simulink model "ar_lht_hw"  (R2018a)
settings: Solver=VariableStepAuto  StartTime=0.0  StopTime=ts*2+2*maxRho*T*2  RelTol=1e-3  EnableMultiTasking=on
PreLoadFcn:
  | currentDir  = pwd;
  | filesepIdx   = strfind(currentDir, filesep);
  | newDir = currentDir(1:filesepIdx(end)-7);
  | 
  | addpath([newDir, '\scripts']);
InitFcn:
  | setup;
  | pre_processing;
StopFcn:
  | post_processing;
  | imtool(O);
values from neighbouring files (symbols this model uses):
  deltaTheta = 1    [setup.m]
  fps = f/((height)*(width))    (= 184.377034505)    [setup.m]
  height = 768    [setup.m]
  K = (maxTheta + deltaTheta)/R    (= 45)    [setup.m]
  maxRho = ceil(sqrt((height/2)^2+(width/2)^2))    [setup.m]
  maxTheta = 179    [setup.m]
  R = 4    [setup.m]
  T = 1/f    (= 6.89655172414e-09)    [setup.m]
  width = 1024    [setup.m]
libraries: xbsIndex_r4 x336, hdlsllib x6, visionhdlutilities x2, visionhdlio x2, simulink x1, dspswit3 x1, visionsources x1
(part 1 of 2)
settings Model: Creator=David Northcote  LastModifiedBy=rgb11127
settings OptimizationCC: LifeSpan=inf
settings DebuggingCC: SFUnexpectedBacktrackingDiag=warning  SFNoUnconditionalDefaultTransitionDiag=warning  SFExecutionAtInitializationDiag=none
settings CodeAppCC: StateflowObjectComments=on
settings GRTTargetCC: TargetLangStandard=C89/C90 (ANSI)  GeneratePreprocessorConditionals=Disable all
settings ConfigComp: CovMetricSettings=dw  CovHtmlReporting=on  CovSaveCumulativeToWorkspaceVar=on  CovSaveSingleToWorkspaceVar=on  CovExternalEMLEnable=off

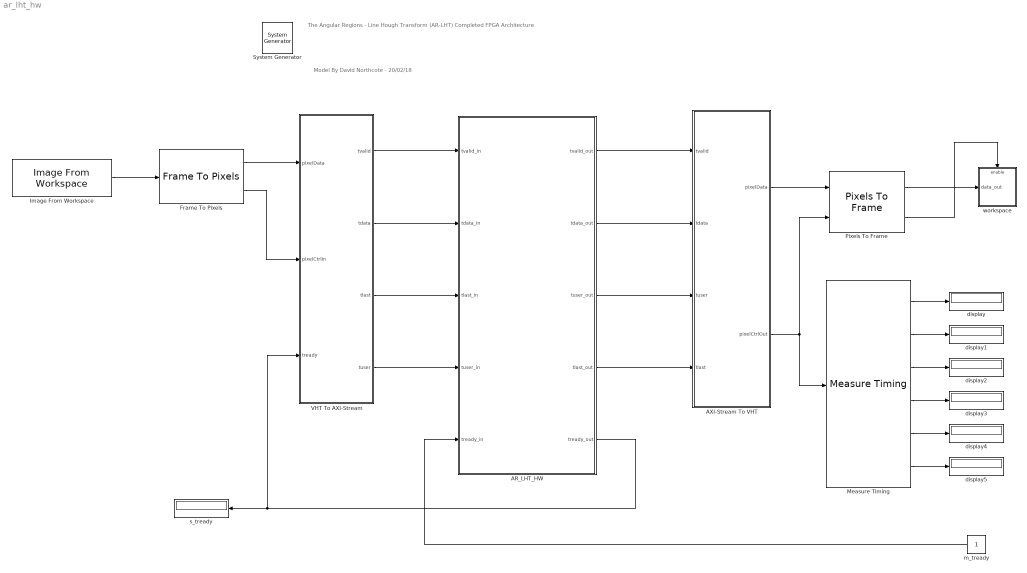
== system ar_lht_hw ==
  note: Model By David Northcote - 20/02/18
  note: The Angular Regions - Line Hough Transform (AR-LHT)
      | Completed FPGA Architecture
  " System Generator" : xbsIndex_r4/ System Generator  Tag=genX  xilinxfamily=zynq  part=xc7z010  speed=-1  package=clg400  synthesis_tool=Vivado  clock_wrapper=Clock Enables  directory=./netlist  proj_type=Vivado  Synth_file=Vivado Synthesis Defaults  Impl_file=Vivado Implementation Defaults  testbench=off  simulink_period=T  sysclk_period=T*1e9  dcm_input_clock_period=10  incr_netlist=off  trim_vbits=Everywhere in SubSystem  dbl_ovrd=According to Block Masks  core_generation=According to Block Masks  run_coregen=off  deprecated_control=off  eval_field=0  block_type=sysgen
  AR_LHT_HW : Subsystem
  AXI-Stream To VHT : Subsystem
  Frame To Pixels : visionhdlio/Frame To Pixels  NumComponents=1  VideoFormat=Custom  ActivePixelsPerLine=width  ActiveVideoLines=height  TotalPixelsPerLine=width  TotalVideoLines=height  StartingActiveLine=1  FrontPorch=0  SampleTime=0
      settings: SourceProductName=Vision HDL Toolbox  SourceProductBaseCode=VT
  Image From Workspace : visionsources/Image From Workspace  Tag=vipblks_nd  ImageValue=InputImage  Ts=1/fps  imagePorts=One multidimensional signal  OutPortLabels=R|G|B  ImageDataType=Inherit from 'Value'  Signed=on  WordLength=16  sdImageDataType=sfix(16)  FractionLengthMode=User-defined  FractionLength=15
      settings: SourceProductName=Computer Vision System Toolbox  SourceProductBaseCode=VP
  Measure Timing : visionhdlutilities/Measure Timing  SimulateUsing=Code generation
      settings: SourceProductName=Vision HDL Toolbox  SourceProductBaseCode=VT
  Pixels To Frame : visionhdlio/Pixels To Frame  NumComponents=1  VideoFormat=Custom  ActivePixelsPerLine=maxRho*2  ActiveVideoLines=maxTheta+deltaTheta  TotalPixelsPerLine=maxRho*2  TotalVideoLines=maxTheta+deltaTheta
      settings: SourceProductName=Vision HDL Toolbox  SourceProductBaseCode=VT
  VHT To AXI-Stream : Subsystem
  display{,1..5} (6 alike) : Display
  m_tready : Constant  OutDataTypeStr=boolean  SampleTime=T
  s_tready : Display
  workspace : Subsystem
  wires:
  Measure Timing/6 -> display5/1
  Measure Timing/5 -> display4/1
  Measure Timing/4 -> display3/1
  Measure Timing/3 -> display2/1
  Measure Timing/2 -> display1/1
  Measure Timing/1 -> display/1
  Pixels To Frame/2 -> workspace/Enable
  Pixels To Frame/1 -> workspace/1(data_out)
  AXI-Stream To VHT/2(pixelCtrlOut) -> Measure Timing/1, Pixels To Frame/2
  AXI-Stream To VHT/1(pixelData) -> Pixels To Frame/1
  Image From Workspace/1 -> Frame To Pixels/1
  Frame To Pixels/2 -> VHT To AXI-Stream/2(pixelCtrlIn)
  Frame To Pixels/1 -> VHT To AXI-Stream/1(pixelData)
  VHT To AXI-Stream/4(tuser) -> AR_LHT_HW/4(tuser_in)
  VHT To AXI-Stream/2(tdata) -> AR_LHT_HW/2(tdata_in)
  VHT To AXI-Stream/3(tlast) -> AR_LHT_HW/3(tlast_in)
  VHT To AXI-Stream/1(tvalid) -> AR_LHT_HW/1(tvalid_in)
  AR_LHT_HW/5(tready_out) -> VHT To AXI-Stream/3(tready), s_tready/1
  AR_LHT_HW/1(tvalid_out) -> AXI-Stream To VHT/1(tvalid)
  AR_LHT_HW/2(tdata_out) -> AXI-Stream To VHT/2(tdata)
  AR_LHT_HW/3(tuser_out) -> AXI-Stream To VHT/3(tuser)
  AR_LHT_HW/4(tlast_out) -> AXI-Stream To VHT/4(tlast)
  m_tready/1 -> AR_LHT_HW/5(tready_in)

== system ar_lht_hw/AR_LHT_HW ==
  tvalid_in : Inport
  tdata_in : Inport  Port=2
  tlast_in : Inport  Port=3
  tuser_in : Inport  Port=4
  tready_in : Inport  Port=5
  DUT : Subsystem
  M_AXIS : Subsystem
  S_AXIS : Subsystem
  tvalid_out : Outport
  tdata_out : Outport  Port=2
  tuser_out : Outport  Port=3
  tlast_out : Outport  Port=4
  tready_out : Outport  Port=5
  wires:
  tdata_in/1 -> S_AXIS/2(tdata_in)
  tuser_in/1 -> S_AXIS/4(tuser_in)
  tvalid_in/1 -> S_AXIS/1(tvalid_in)
  tlast_in/1 -> S_AXIS/3(tlast_in)
  M_AXIS/2(tvalid_out) -> tvalid_out/1
  tready_in/1 -> M_AXIS/5(tready_in)
  M_AXIS/3(tdata_out) -> tdata_out/1
  M_AXIS/5(tlast_out) -> tlast_out/1
  S_AXIS/5(tready_out) -> tready_out/1
  M_AXIS/4(tuser_out) -> tuser_out/1
  S_AXIS/4(tuser_out) -> DUT/4(tuser_in)
  S_AXIS/3(tlast_out) -> DUT/3(tlast_in)
  S_AXIS/1(tvalid_out) -> DUT/1(tvalid_in)
  S_AXIS/2(tdata_out) -> DUT/2(tdata_in)
  DUT/4(tuser_out) -> M_AXIS/4(tuser_in)
  DUT/3(tlast_out) -> M_AXIS/3(tlast_in)
  DUT/2(tdata_out) -> M_AXIS/2(tdata_in)
  DUT/1(tvalid_out) -> M_AXIS/1(tvalid_in)
  M_AXIS/1(tready_out) -> DUT/5(tready_in)
  DUT/5(tready_out) -> S_AXIS/5(tready_in)

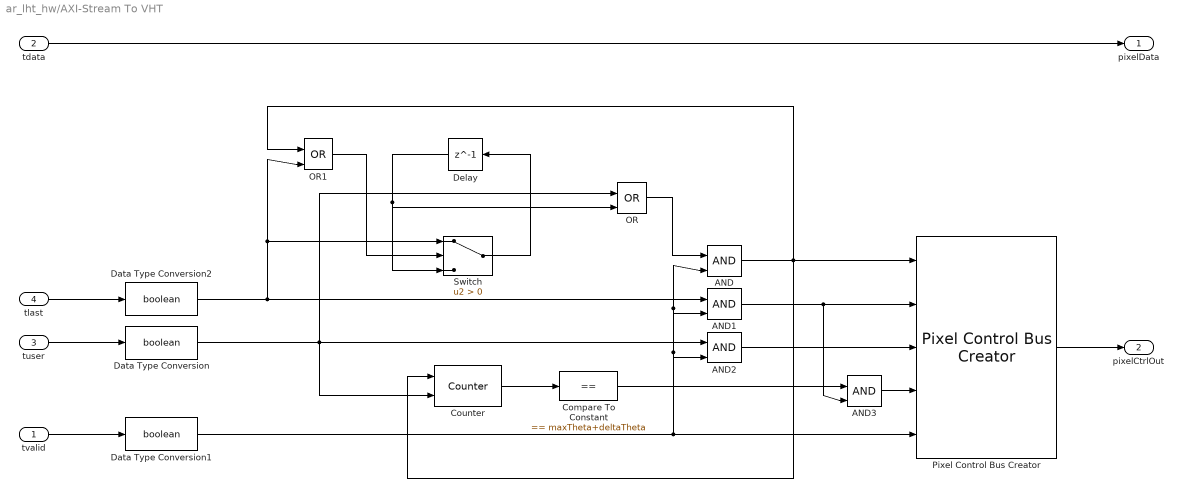
== system ar_lht_hw/AXI-Stream To VHT ==
  tvalid : Inport
  tdata : Inport  Port=2
  tuser : Inport  Port=3
  tlast : Inport  Port=4
  AND{,1..3} (4 alike) : Logic  IconShape=distinctive  AllPortsSameDT=off  OutDataTypeStr=boolean
  Compare To Constant : simulink/Logic and Bit Operations/Compare To Constant  relop===  const=maxTheta+deltaTheta  OutDataTypeStr=boolean
  Counter : dspswit3/Counter  Direction=Up  CountEvent=Non-zero sample  CounterSize=32 bits  MaxCount=255  InitialCount=0  Output=Count  HitValue=32  ResetInput=on  SamplesPerFrame=1  Ts=1  CntDtype=uint32  HitDtype=Logical
  Data Type Conversion : DataTypeConversion  OutDataTypeStr=boolean
  Data Type Conversion1 : DataTypeConversion  OutDataTypeStr=boolean
  Data Type Conversion2 : DataTypeConversion  OutDataTypeStr=boolean
  Delay : Delay  DelayLength=1
  OR : Logic  Operator=OR  IconShape=distinctive  AllPortsSameDT=off  OutDataTypeStr=boolean
  OR1 : Logic  Operator=OR  IconShape=distinctive  AllPortsSameDT=off  OutDataTypeStr=boolean
  Pixel Control Bus Creator : visionhdlutilities/Pixel Control Bus Creator
      settings: SourceProductName=Vision HDL Toolbox  SourceProductBaseCode=VT
  Switch : Switch  Criteria=u2 > Threshold
  pixelData : Outport
  pixelCtrlOut : Outport  Port=2
  wires:
  AND3/1 -> Pixel Control Bus Creator/4
  AND1/1 -> Pixel Control Bus Creator/2, AND3/2
  Compare To Constant/1 -> AND3/1
  AND2/1 -> Pixel Control Bus Creator/3
  AND/1 -> Pixel Control Bus Creator/1, OR1/1, Counter/1
  OR1/1 -> Switch/2
  Delay/1 -> Switch/3, OR/2
  Switch/1 -> Delay/1
  OR/1 -> AND/1
  Data Type Conversion/1 -> OR/1, AND2/1, Counter/2
  Data Type Conversion1/1 -> Pixel Control Bus Creator/5, AND/2, AND1/2, AND2/2
  Data Type Conversion2/1 -> Switch/1, OR1/2, AND1/1
  Counter/1 -> Compare To Constant/1
  tvalid/1 -> Data Type Conversion1/1
  tlast/1 -> Data Type Conversion2/1
  tuser/1 -> Data Type Conversion/1
  Pixel Control Bus Creator/1 -> pixelCtrlOut/1
  tdata/1 -> pixelData/1

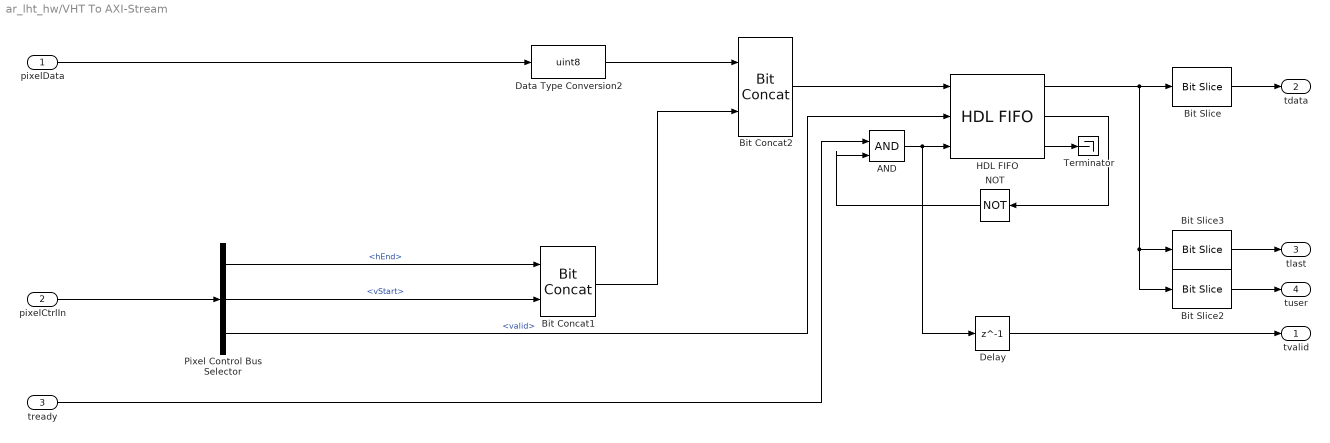
== system ar_lht_hw/VHT To AXI-Stream ==
  pixelData : Inport
  pixelCtrlIn : Inport  Port=2
  tready : Inport  Port=3
  AND : Logic  IconShape=distinctive  AllPortsSameDT=off  OutDataTypeStr=boolean
  Bit Concat1 : hdlsllib/Logic and Bit Operations/Bit Concat  numInputs=2
      settings: SourceProductName=HDL Coder  SourceProductBaseCode=HD
  Bit Concat2 : hdlsllib/Logic and Bit Operations/Bit Concat  numInputs=2
      settings: SourceProductName=HDL Coder  SourceProductBaseCode=HD
  Bit Slice : hdlsllib/Logic and Bit Operations/Bit Slice  lidx=9  ridx=2
  Bit Slice2 : hdlsllib/Logic and Bit Operations/Bit Slice  lidx=0  ridx=0
  Bit Slice3 : hdlsllib/Logic and Bit Operations/Bit Slice  lidx=1  ridx=1
  Data Type Conversion2 : DataTypeConversion  OutDataTypeStr=uint8
  Delay : Delay  DelayLength=1
  HDL FIFO : hdlsllib/HDL RAMs/HDL FIFO  fifo_size=1024  ratio=1  push_msg=Error  pop_msg=Error  show_empty=on  show_full=on  show_num=off
      settings: SourceProductName=HDL Coder  SourceProductBaseCode=HD
  NOT : Logic  Operator=NOT  IconShape=distinctive  AllPortsSameDT=off  OutDataTypeStr=boolean
  Pixel Control Bus Selector : BusSelector  OutputSignals=hEnd,vStart,valid
  Terminator : Terminator
  tvalid : Outport
  tdata : Outport  Port=2
  tlast : Outport  Port=3
  tuser : Outport  Port=4
  wires:
  HDL FIFO/3 -> Terminator/1
  Delay/1 -> tvalid/1
  Pixel Control Bus Selector/3 -> HDL FIFO/2  "<valid>"
  Pixel Control Bus Selector/2 -> Bit Concat1/2  "<vStart>"
  Pixel Control Bus Selector/1 -> Bit Concat1/1  "<hEnd>"
  AND/1 -> HDL FIFO/3, Delay/1
  Bit Slice2/1 -> tuser/1
  Bit Slice3/1 -> tlast/1
  Bit Slice/1 -> tdata/1
  NOT/1 -> AND/2
  HDL FIFO/2 -> NOT/1
  tready/1 -> AND/1
  HDL FIFO/1 -> Bit Slice/1, Bit Slice2/1, Bit Slice3/1
  Bit Concat1/1 -> Bit Concat2/2
  Data Type Conversion2/1 -> Bit Concat2/1
  Bit Concat2/1 -> HDL FIFO/1
  pixelCtrlIn/1 -> Pixel Control Bus Selector/1
  pixelData/1 -> Data Type Conversion2/1

== system ar_lht_hw/workspace ==
  data_out : Inport
  Enable : EnablePort
  To Workspace : ToWorkspace  VariableName=data_out  SampleTime=-1
      settings: MaxDataPoints=1
  wires:
  data_out/1 -> To Workspace/1

== system ar_lht_hw/AR_LHT_HW/DUT ==
  tvalid_in : Inport
  tdata_in : Inport  Port=2
  tlast_in : Inport  Port=3
  tuser_in : Inport  Port=4
  tready_in : Inport  Port=5
  AXI FIFO : xbsIndex_r4/AXI FIFO  input_depth_axis=16  actual_fifo_depth_label=18  enable_tdata=on  enable_tdest=off  enable_tstrb=off  enable_tready=on  enable_tid=off  enable_tuser=on  enable_tkeep=off  enable_tlast=on  has_aresetn=off  enable_data_counts_axis=off  fifo_implementation_type_axis=Common Clock Distributed RAM  trim_axipin_name=on  programmable_full_type_axis=Full  full_threshold_assert_value_axis=0  programmable_empty_type_axis=Empty  empty_threshold_assert_value_axis=1022  underflow_flag_axi=0  underflow_sense_axi=Active High  overflow_flag_axi=0  overflow_sense_axi=Active High  block_type=axi_fifo
  Algorithm : Subsystem
  tvalid_out : Outport
  tdata_out : Outport  Port=2
  tlast_out : Outport  Port=3
  tuser_out : Outport  Port=4
  tready_out : Outport  Port=5
  wires:
  Algorithm/1(tready_out) -> AXI FIFO/1
  Algorithm/2(tvalid_out) -> AXI FIFO/2
  Algorithm/3(tdata_out) -> AXI FIFO/3
  Algorithm/4(tlast_out) -> AXI FIFO/4
  Algorithm/5(tuser_out) -> AXI FIFO/5
  AXI FIFO/5 -> tready_out/1
  AXI FIFO/2 -> tdata_out/1
  AXI FIFO/1 -> tvalid_out/1
  AXI FIFO/3 -> tlast_out/1
  AXI FIFO/4 -> tuser_out/1
  tdata_in/1 -> Algorithm/3(tdata_in)
  tuser_in/1 -> Algorithm/5(tuser_in)
  tlast_in/1 -> Algorithm/4(tlast_in)
  tready_in/1 -> Algorithm/1(tready_in)
  tvalid_in/1 -> Algorithm/2(tvalid_in)

== system ar_lht_hw/AR_LHT_HW/M_AXIS ==
  tvalid_in : Inport
  tdata_in : Inport  Port=2
  tlast_in : Inport  Port=3
  tuser_in : Inport  Port=4
  tready_in : Inport  Port=5
  m_axis_tdata : xbsIndex_r4/Gateway Out  inherit_from_input=on  hdl_port=on  rows=1  columns=1  UseAsDAC=off  DACChannel='1'  interface=None  automatic_assignment=on  address_offset=hex2dec('00')  intf_name=''  intf_description=''  timing_constraint=None  locs_specified=off  LOCs={}  io_standard={}  block_type=gatewayout
  m_axis_tlast : xbsIndex_r4/Gateway Out  inherit_from_input=off  hdl_port=on  rows=1  columns=1  UseAsDAC=off  DACChannel='1'  interface=None  automatic_assignment=on  address_offset=hex2dec('00')  intf_name=''  intf_description=''  timing_constraint=None  locs_specified=off  LOCs={}  io_standard={}  block_type=gatewayout
  m_axis_tready : xbsIndex_r4/Gateway In  gui_display_data_type=Boolean  arith_type=Boolean  n_bits=16  bin_pt=14  preci_type=Single  exp_width=8  frac_width=24  rows=1  columns=1  quantization="Round  (unbiased: +/- Inf)"  overflow=Saturate  period=T  UseAsADC=off  ADCChannel='1'  interface=None  automatic_assignment=on  address_offset=hex2dec('00')  intf_name=''  intf_description=''  default_value=0  timing_constraint=None  locs_specified=off  LOCs={}  io_standard={}  inherit_from_input=off  hdl_port=on  dbl_ovrd=off  block_type=gatewayin
  m_axis_tuser : xbsIndex_r4/Gateway Out  inherit_from_input=off  hdl_port=on  rows=1  columns=1  UseAsDAC=off  DACChannel='1'  interface=None  automatic_assignment=on  address_offset=hex2dec('00')  intf_name=''  intf_description=''  timing_constraint=None  locs_specified=off  LOCs={}  io_standard={}  block_type=gatewayout
  m_axis_tvalid : xbsIndex_r4/Gateway Out  inherit_from_input=off  hdl_port=on  rows=1  columns=1  UseAsDAC=off  DACChannel='1'  interface=None  automatic_assignment=on  address_offset=hex2dec('00')  intf_name=''  intf_description=''  timing_constraint=None  locs_specified=off  LOCs={}  io_standard={}  block_type=gatewayout
  tready_out : Outport
  tvalid_out : Outport  Port=2
  tdata_out : Outport  Port=3
  tuser_out : Outport  Port=4
  tlast_out : Outport  Port=5
  wires:
  m_axis_tuser/1 -> tuser_out/1
  m_axis_tvalid/1 -> tvalid_out/1
  m_axis_tdata/1 -> tdata_out/1
  tready_in/1 -> m_axis_tready/1
  tvalid_in/1 -> m_axis_tvalid/1
  m_axis_tlast/1 -> tlast_out/1
  tdata_in/1 -> m_axis_tdata/1
  tlast_in/1 -> m_axis_tlast/1
  m_axis_tready/1 -> tready_out/1
  tuser_in/1 -> m_axis_tuser/1

== system ar_lht_hw/AR_LHT_HW/S_AXIS ==
  tvalid_in : Inport
  tdata_in : Inport  Port=2
  tlast_in : Inport  Port=3
  tuser_in : Inport  Port=4
  tready_in : Inport  Port=5
  s_axis_tdata : xbsIndex_r4/Gateway In  gui_display_data_type=Fixed-point  arith_type=Unsigned  n_bits=8  bin_pt=0  preci_type=Single  exp_width=8  frac_width=24  rows=1  columns=1  quantization=Truncate  overflow=Flag as error  period=T  UseAsADC=off  ADCChannel='1'  interface=None  automatic_assignment=on  address_offset=hex2dec('00')  intf_name=''  intf_description=''  default_value=0  timing_constraint=None  locs_specified=off  LOCs={}  io_standard={}  inherit_from_input=off  hdl_port=on  dbl_ovrd=off  block_type=gatewayin
  s_axis_tlast : xbsIndex_r4/Gateway In  gui_display_data_type=Boolean  arith_type=Boolean  n_bits=32  bin_pt=0  preci_type=Single  exp_width=8  frac_width=24  rows=1  columns=1  quantization=Truncate  overflow=Flag as error  period=T  UseAsADC=off  ADCChannel='1'  interface=None  automatic_assignment=on  address_offset=hex2dec('00')  intf_name=''  intf_description=''  default_value=0  timing_constraint=None  locs_specified=off  LOCs={}  io_standard={}  inherit_from_input=off  hdl_port=on  dbl_ovrd=off  block_type=gatewayin
  s_axis_tready : xbsIndex_r4/Gateway Out  inherit_from_input=on  hdl_port=on  rows=1  columns=1  UseAsDAC=off  DACChannel='1'  interface=None  automatic_assignment=on  address_offset=hex2dec('00')  intf_name=''  intf_description=''  timing_constraint=None  locs_specified=off  LOCs={}  io_standard={}  block_type=gatewayout
  s_axis_tuser : xbsIndex_r4/Gateway In  gui_display_data_type=Boolean  arith_type=Boolean  n_bits=1  bin_pt=0  preci_type=Single  exp_width=8  frac_width=24  rows=1  columns=1  quantization=Truncate  overflow=Flag as error  period=T  UseAsADC=off  ADCChannel='1'  interface=None  automatic_assignment=on  address_offset=hex2dec('00')  intf_name=''  intf_description=''  default_value=0  timing_constraint=None  locs_specified=off  LOCs={}  io_standard={}  inherit_from_input=off  hdl_port=on  dbl_ovrd=off  block_type=gatewayin
  s_axis_tvalid : xbsIndex_r4/Gateway In  gui_display_data_type=Boolean  arith_type=Boolean  n_bits=32  bin_pt=0  preci_type=Single  exp_width=8  frac_width=24  rows=1  columns=1  quantization=Truncate  overflow=Flag as error  period=T  UseAsADC=off  ADCChannel='1'  interface=None  automatic_assignment=on  address_offset=hex2dec('00')  intf_name=''  intf_description=''  default_value=0  timing_constraint=None  locs_specified=off  LOCs={}  io_standard={}  inherit_from_input=off  hdl_port=on  dbl_ovrd=off  block_type=gatewayin
  tvalid_out : Outport
  tdata_out : Outport  Port=2
  tlast_out : Outport  Port=3
  tuser_out : Outport  Port=4
  tready_out : Outport  Port=5
  wires:
  s_axis_tready/1 -> tready_out/1
  tready_in/1 -> s_axis_tready/1
  tuser_in/1 -> s_axis_tuser/1
  tlast_in/1 -> s_axis_tlast/1
  tvalid_in/1 -> s_axis_tvalid/1
  tdata_in/1 -> s_axis_tdata/1
  s_axis_tvalid/1 -> tvalid_out/1
  s_axis_tdata/1 -> tdata_out/1
  s_axis_tlast/1 -> tlast_out/1
  s_axis_tuser/1 -> tuser_out/1

== system ar_lht_hw/AR_LHT_HW/DUT/Algorithm ==
  note: tready should never have any latency. It will only be used to pop the IP core's front-end FIFO.
  tready_in : Inport
  tvalid_in : Inport  Port=2
  tdata_in : Inport  Port=3
  tlast_in : Inport  Port=4
  tuser_in : Inport  Port=5
  AlgorithmDUT_ARHough : Subsystem
  AlgorithmDUT_Open : Subsystem
  tready_out : Outport
  tvalid_out : Outport  Port=2
  tdata_out : Outport  Port=3
  tlast_out : Outport  Port=4
  tuser_out : Outport  Port=5
  wires:
  tready_in/1 -> tready_out/1
  tvalid_in/1 -> AlgorithmDUT_ARHough/4(tvalid_in)
  tuser_in/1 -> AlgorithmDUT_ARHough/1(tuser_in)
  tlast_in/1 -> AlgorithmDUT_ARHough/2(tlast_in)
  tdata_in/1 -> AlgorithmDUT_ARHough/3(tdata_in)
  AlgorithmDUT_ARHough/1(tuser_out) -> AlgorithmDUT_Open/1(tuser_in)
  AlgorithmDUT_ARHough/2(tlast_out) -> AlgorithmDUT_Open/2(tlast_in)
  AlgorithmDUT_ARHough/3(tdata_out) -> AlgorithmDUT_Open/3(tdata_in)
  AlgorithmDUT_ARHough/4(tvalid_out) -> AlgorithmDUT_Open/4(tvalid_in)
  AlgorithmDUT_Open/1(tuser_out) -> tuser_out/1
  AlgorithmDUT_Open/2(tlast_out) -> tlast_out/1
  AlgorithmDUT_Open/3(tdata_out) -> tdata_out/1
  AlgorithmDUT_Open/4(tvalid_out) -> tvalid_out/1

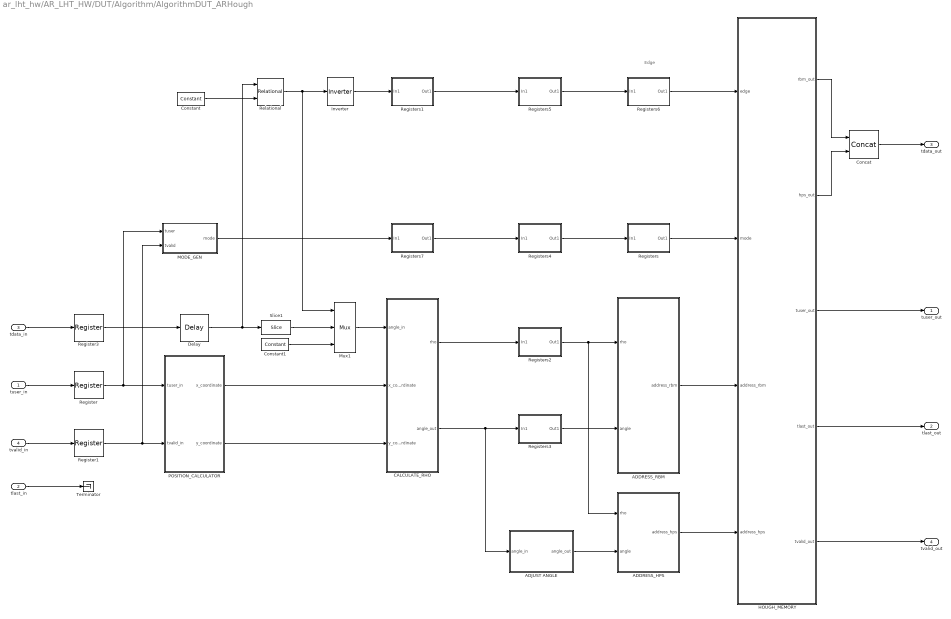
== system ar_lht_hw/AR_LHT_HW/DUT/Algorithm/AlgorithmDUT_ARHough ==
  note: Edge
  tuser_in : Inport
  tlast_in : Inport  Port=2
  tdata_in : Inport  Port=3
  tvalid_in : Inport  Port=4
  ADDRESS_HPS : Subsystem
  ADDRESS_RBM : Subsystem
  ADJUST ANGLE : Subsystem
  CALCULATE_RHO : Subsystem
  Concat : xbsIndex_r4/Concat  num_inputs=2  dbl_ovrd=off  block_type=concat
  Constant : xbsIndex_r4/Constant  const=255  gui_display_data_type=Fixed-point  arith_type=Unsigned  n_bits=8  bin_pt=0  preci_type=Single  exp_width=8  frac_width=24  explicit_period=on  period=T  equ=P=C  opselect=C  inp2=PCIN>>17  opr=+  inp1=P  carry=CIN  dbl_ovrd=off  block_type=constant
  Constant1 : xbsIndex_r4/Constant  const=0  gui_display_data_type=Fixed-point  arith_type=Unsigned  n_bits=8  bin_pt=0  preci_type=Single  exp_width=8  frac_width=24  explicit_period=on  period=T  equ=P=C  opselect=C  inp2=PCIN>>17  opr=+  inp1=P  carry=CIN  dbl_ovrd=off  block_type=constant
  Delay : xbsIndex_r4/Delay  rst=off  infoeditControl=Selection of Reset will increase slice count due to use of real FFs and instead of SRLs  en=off  latency=1  reg_retiming=off  dbl_ovrd=off  block_type=delay
  HOUGH_MEMORY : Subsystem
  Inverter : xbsIndex_r4/Inverter  en=off  latency=0  dbl_ovrd=off  block_type=inv
  MODE_GEN : Subsystem
  Mux1 : xbsIndex_r4/Mux  inputs=2  en=off  latency=0  precision=Full  arith_type=Unsigned  n_bits=16  bin_pt=14  quantization=Truncate  overflow=Wrap  dbl_ovrd=off  block_type=mux
  POSITION_CALCULATOR : Subsystem
  Register : xbsIndex_r4/Register  init=0  rst=off  en=off  dbl_ovrd=off  block_type=register
  Register1 : xbsIndex_r4/Register  init=0  rst=off  en=off  dbl_ovrd=off  block_type=register
  Register3 : xbsIndex_r4/Register  init=0  rst=off  en=off  dbl_ovrd=off  block_type=register
  Registers : Subsystem
  Registers1 : Subsystem
  Registers2 : Subsystem
  Registers3 : Subsystem
  Registers4 : Subsystem
  Registers5 : Subsystem
  Registers6 : Subsystem
  Registers7 : Subsystem
  Relational : xbsIndex_r4/Relational  mode=a=b  op_type=Bool  en=off  latency=0  dbl_ovrd=off  block_type=relational
  Slice1 : xbsIndex_r4/Slice  nbits=8  boolean_output=off  mode=Two Bit Locations  bit1=7  base1=LSB of Input  bit0=0  base0=LSB of Input  dbl_ovrd=off  block_type=slice
  Terminator : Terminator
  tuser_out : Outport
  tlast_out : Outport  Port=2
  tdata_out : Outport  Port=3
  tvalid_out : Outport  Port=4
  wires:
  Delay/1 -> Relational/1, Slice1/1
  Registers1/1(Out1) -> Registers5/1(In1)
  Registers5/1(Out1) -> Registers6/1(In1)
  Relational/1 -> Mux1/1, Inverter/1
  Register3/1 -> Delay/1
  Register/1 -> MODE_GEN/1(tuser), POSITION_CALCULATOR/1(tuser_in)
  CALCULATE_RHO/1(rho) -> Registers2/1(In1)
  Registers2/1(Out1) -> ADDRESS_RBM/1(rho), ADDRESS_HPS/1(rho)
  Registers3/1(Out1) -> ADDRESS_RBM/2(angle)
  ADJUST ANGLE/1(angle_out) -> ADDRESS_HPS/2(angle)
  CALCULATE_RHO/2(angle_out) -> Registers3/1(In1), ADJUST ANGLE/1(angle_in)
  POSITION_CALCULATOR/1(x_coordinate) -> CALCULATE_RHO/2(x_coordinate)
  POSITION_CALCULATOR/2(y_coordinate) -> CALCULATE_RHO/3(y_coordinate)
  tlast_in/1 -> Terminator/1
  Constant/1 -> Relational/2
  Mux1/1 -> CALCULATE_RHO/1(angle_in)
  Slice1/1 -> Mux1/2
  Constant1/1 -> Mux1/3
  Inverter/1 -> Registers1/1(In1)
  MODE_GEN/1(mode) -> Registers7/1(In1)
  Registers7/1(Out1) -> Registers4/1(In1)
  Registers4/1(Out1) -> Registers/1(In1)
  Register1/1 -> MODE_GEN/2(tvalid), POSITION_CALCULATOR/2(tvalid_in)
  Registers6/1(Out1) -> HOUGH_MEMORY/1(edge)
  Registers/1(Out1) -> HOUGH_MEMORY/2(mode)
  ADDRESS_RBM/1(address_rbm) -> HOUGH_MEMORY/3(address_rbm)
  ADDRESS_HPS/1(address_hps) -> HOUGH_MEMORY/4(address_hps)
  HOUGH_MEMORY/2(hps_out) -> Concat/2
  HOUGH_MEMORY/1(rbm_out) -> Concat/1
  HOUGH_MEMORY/5(tvalid_out) -> tvalid_out/1
  tvalid_in/1 -> Register1/1
  tuser_in/1 -> Register/1
  tdata_in/1 -> Register3/1
  HOUGH_MEMORY/4(tlast_out) -> tlast_out/1
  HOUGH_MEMORY/3(tuser_out) -> tuser_out/1
  Concat/1 -> tdata_out/1

== system ar_lht_hw/AR_LHT_HW/DUT/Algorithm/AlgorithmDUT_Open ==
  tuser_in : Inport
  tlast_in : Inport  Port=2
  tdata_in : Inport  Port=3
  tvalid_in : Inport  Port=4
  Clear2 : xbsIndex_r4/Constant  const=0  gui_display_data_type=Fixed-point  arith_type=Unsigned  n_bits=18  bin_pt=0  preci_type=Single  exp_width=8  frac_width=24  explicit_period=on  period=T  equ=P=C  opselect=C  inp2=PCIN>>17  opr=+  inp1=P  carry=CIN  dbl_ovrd=off  block_type=constant
  Delay2 : xbsIndex_r4/Delay  rst=off  infoeditControl=Selection of Reset will increase slice count due to use of real FFs and instead of SRLs  en=off  latency=(2*maxRho+1)*2+3  reg_retiming=off  dbl_ovrd=off  block_type=delay
  MorphoOpen : Subsystem  mask{width=2*maxRho, height=maxTheta+deltaTheta}
      mask prompts: width "Enter image width."; height "Enter image height."
  Mux3 : xbsIndex_r4/Mux  inputs=2  en=off  latency=0  precision=Full  arith_type=Unsigned  n_bits=16  bin_pt=14  quantization=Truncate  overflow=Wrap  dbl_ovrd=off  block_type=mux
  hps : xbsIndex_r4/Slice  nbits=1  boolean_output=off  mode=Two Bit Locations  bit1=17  base1=LSB of Input  bit0=0  base0=LSB of Input  dbl_ovrd=off  block_type=slice
  msb : xbsIndex_r4/Slice  nbits=1  boolean_output=on  mode=Upper Bit Location + Width  bit1=0  base1=MSB of Input  bit0=0  base0=LSB of Input  dbl_ovrd=off  block_type=slice
  tuser_out : Outport
  tlast_out : Outport  Port=2
  tdata_out : Outport  Port=3
  tvalid_out : Outport  Port=4
  wires:
  tdata_in/1 -> msb/1, hps/1
  Delay2/1 -> Mux3/3
  Clear2/1 -> Mux3/2
  MorphoOpen/4(tvalid_out) -> tvalid_out/1
  MorphoOpen/3(tdata_out) -> Mux3/1
  MorphoOpen/1(tuser_out) -> tuser_out/1
  MorphoOpen/2(tlast_out) -> tlast_out/1
  Mux3/1 -> tdata_out/1
  hps/1 -> Delay2/1
  msb/1 -> MorphoOpen/3(tdata_in)
  tlast_in/1 -> MorphoOpen/2(tlast_in)
  tuser_in/1 -> MorphoOpen/1(tuser_in)
  tvalid_in/1 -> MorphoOpen/4(tvalid_in)

== system ar_lht_hw/AR_LHT_HW/DUT/Algorithm/AlgorithmDUT_ARHough/ADDRESS_HPS ==
  rho : Inport
  angle : Inport  Port=2
  AddSub1 : xbsIndex_r4/AddSub  mode=Addition  use_carryin=off  use_carryout=off  en=off  latency=1  precision=User Defined  arith_type=Unsigned  n_bits=ceil(log2(maxRho*2))  bin_pt=0  quantization=Truncate  overflow=Wrap  use_behavioral_HDL=on  hw_selection=Fabric  pipelined=on  dbl_ovrd=off  block_type=addsub
  AddSub2 : xbsIndex_r4/AddSub  mode=Addition  use_carryin=off  use_carryout=off  en=off  latency=1  precision=User Defined  arith_type=Unsigned  n_bits=ceil(log2(maxRho*2)+log2(K-1))  bin_pt=0  quantization=Truncate  overflow=Wrap  use_behavioral_HDL=on  hw_selection=Fabric  pipelined=on  dbl_ovrd=off  block_type=addsub
  CMult : xbsIndex_r4/CMult  const=maxRho*2  gui_display_data_type=Fixed-point  const_n_bits=ceil(log2(maxRho)+1)  const_bin_pt=0  float_type=Single  exp_bits=8  fraction_bits=24  en=off  latency=1  precision=Full  arith_type="Signed  (2's comp)"  n_bits=16  bin_pt=14  quantization=Truncate  overflow=Wrap  use_behavioral_HDL=off  mem_type=Distributed RAM  pipeline=off  dbl_ovrd=off  block_type=cmult
  rho_offset_general : xbsIndex_r4/Constant  const=maxRho-1  gui_display_data_type=Fixed-point  arith_type=Unsigned  n_bits=ceil(log2(maxRho-1))  bin_pt=0  preci_type=Single  exp_width=8  frac_width=24  explicit_period=on  period=T  equ=P=C  opselect=C  inp2=PCIN>>17  opr=+  inp1=P  carry=CIN  dbl_ovrd=off  block_type=constant
  address_hps : Outport
  wires:
  CMult/1 -> AddSub2/2
  AddSub2/1 -> address_hps/1
  angle/1 -> CMult/1
  rho_offset_general/1 -> AddSub1/1
  AddSub1/1 -> AddSub2/1
  rho/1 -> AddSub1/2

== system ar_lht_hw/AR_LHT_HW/DUT/Algorithm/AlgorithmDUT_ARHough/ADDRESS_RBM ==
  rho : Inport
  angle : Inport  Port=2
  AddSub1 : xbsIndex_r4/AddSub  mode=Addition  use_carryin=off  use_carryout=off  en=off  latency=1  precision=User Defined  arith_type=Unsigned  n_bits=ceil(log2(maxRho*2))  bin_pt=0  quantization=Truncate  overflow=Saturate  use_behavioral_HDL=on  hw_selection=Fabric  pipelined=on  dbl_ovrd=off  block_type=addsub
  AddSub2 : xbsIndex_r4/AddSub  mode=Addition  use_carryin=off  use_carryout=off  en=off  latency=1  precision=User Defined  arith_type=Unsigned  n_bits=ceil(log2(maxRho*2)+log2(maxTheta))  bin_pt=0  quantization=Truncate  overflow=Wrap  use_behavioral_HDL=on  hw_selection=Fabric  pipelined=on  dbl_ovrd=off  block_type=addsub
  CMult : xbsIndex_r4/CMult  const=maxRho*2  gui_display_data_type=Fixed-point  const_n_bits=ceil(log2(maxRho)+1)  const_bin_pt=0  float_type=Single  exp_bits=8  fraction_bits=24  en=off  latency=1  precision=Full  arith_type="Signed  (2's comp)"  n_bits=16  bin_pt=14  quantization=Truncate  overflow=Wrap  use_behavioral_HDL=off  mem_type=Distributed RAM  pipeline=off  dbl_ovrd=off  block_type=cmult
  rho_offset_general : xbsIndex_r4/Constant  const=maxRho-1  gui_display_data_type=Fixed-point  arith_type=Unsigned  n_bits=ceil(log2(maxRho-1))  bin_pt=0  preci_type=Single  exp_width=8  frac_width=24  explicit_period=on  period=T  equ=P=C  opselect=C  inp2=PCIN>>17  opr=+  inp1=P  carry=CIN  dbl_ovrd=off  block_type=constant
  address_rbm : Outport
  wires:
  rho/1 -> AddSub1/2
  AddSub1/1 -> AddSub2/1
  rho_offset_general/1 -> AddSub1/1
  angle/1 -> CMult/1
  AddSub2/1 -> address_rbm/1
  CMult/1 -> AddSub2/2

== system ar_lht_hw/AR_LHT_HW/DUT/Algorithm/AlgorithmDUT_ARHough/ADJUST ANGLE ==
  angle_in : Inport
  AddSub : xbsIndex_r4/AddSub  mode=Subtraction  use_carryin=off  use_carryout=off  en=off  latency=1  precision=Full  arith_type=Unsigned  n_bits=16  bin_pt=14  quantization=Truncate  overflow=Wrap  use_behavioral_HDL=off  hw_selection=Fabric  pipelined=off  dbl_ovrd=off  block_type=addsub
  AddSub1 : xbsIndex_r4/AddSub  mode=Addition  use_carryin=off  use_carryout=off  en=off  latency=1  precision=Full  arith_type=Unsigned  n_bits=16  bin_pt=14  quantization=Truncate  overflow=Wrap  use_behavioral_HDL=off  hw_selection=Fabric  pipelined=off  dbl_ovrd=off  block_type=addsub
  AddSub2 : xbsIndex_r4/AddSub  mode=Addition  use_carryin=off  use_carryout=off  en=off  latency=1  precision=Full  arith_type=Unsigned  n_bits=16  bin_pt=14  quantization=Truncate  overflow=Wrap  use_behavioral_HDL=off  hw_selection=Fabric  pipelined=off  dbl_ovrd=off  block_type=addsub
  Constant1 : xbsIndex_r4/Constant  const=K-deltaTheta  gui_display_data_type=Fixed-point  arith_type=Unsigned  n_bits=ceil(log2(K-deltaTheta))  bin_pt=0  preci_type=Single  exp_width=8  frac_width=24  explicit_period=on  period=T  equ=P=C  opselect=C  inp2=PCIN>>17  opr=+  inp1=P  carry=CIN  dbl_ovrd=off  block_type=constant
  Constant2 : xbsIndex_r4/Constant  const=maxTheta + deltaTheta - K  gui_display_data_type=Fixed-point  arith_type=Unsigned  n_bits=ceil(log2(maxTheta - K))  bin_pt=0  preci_type=Single  exp_width=8  frac_width=24  explicit_period=on  period=T  equ=P=C  opselect=C  inp2=PCIN>>17  opr=+  inp1=P  carry=CIN  dbl_ovrd=off  block_type=constant
  Constant3 : xbsIndex_r4/Constant  const=K  gui_display_data_type=Fixed-point  arith_type=Unsigned  n_bits=ceil(log2(K))  bin_pt=0  preci_type=Single  exp_width=8  frac_width=24  explicit_period=on  period=T  equ=P=C  opselect=C  inp2=PCIN>>17  opr=+  inp1=P  carry=CIN  dbl_ovrd=off  block_type=constant
  Convert : xbsIndex_r4/Convert  gui_display_data_type=Fixed-point  arith_type=Unsigned  n_bits=ceil(log2(K-deltaTheta))  bin_pt=0  float_type=Single  exp_bits=8  fraction_bits=24  quantization=Truncate  overflow=Wrap  en=off  latency=0  pipeline=off  dbl_ovrd=off  block_type=convert
  MSB : xbsIndex_r4/Slice  nbits=8  boolean_output=on  mode=Upper Bit Location + Width  bit1=0  base1=MSB of Input  bit0=24  base0=LSB of Input  dbl_ovrd=off  block_type=slice
  MSB1 : xbsIndex_r4/Slice  nbits=8  boolean_output=on  mode=Upper Bit Location + Width  bit1=0  base1=MSB of Input  bit0=24  base0=LSB of Input  dbl_ovrd=off  block_type=slice
  Mux1 : xbsIndex_r4/Mux  inputs=2  en=off  latency=0  precision=Full  arith_type=Unsigned  n_bits=16  bin_pt=14  quantization=Truncate  overflow=Wrap  dbl_ovrd=off  block_type=mux
  Mux2 : xbsIndex_r4/Mux  inputs=2  en=off  latency=0  precision=Full  arith_type=Unsigned  n_bits=16  bin_pt=14  quantization=Truncate  overflow=Wrap  dbl_ovrd=off  block_type=mux
  Mux3 : xbsIndex_r4/Mux  inputs=2  en=off  latency=0  precision=Full  arith_type=Unsigned  n_bits=16  bin_pt=14  quantization=Truncate  overflow=Wrap  dbl_ovrd=off  block_type=mux
  Register10 : xbsIndex_r4/Register  init=0  rst=off  en=off  dbl_ovrd=off  block_type=register
  Register11 : xbsIndex_r4/Register  init=0  rst=off  en=off  dbl_ovrd=off  block_type=register
  Register9 : xbsIndex_r4/Register  init=0  rst=off  en=off  dbl_ovrd=off  block_type=register
  Relational : xbsIndex_r4/Relational  mode=a>b  op_type=Bool  en=off  latency=1  dbl_ovrd=off  block_type=relational
  angle_out : Outport
  wires:
  Convert/1 -> angle_out/1
  Register9/1 -> Mux1/2
  Constant2/1 -> AddSub/2
  Constant3/1 -> AddSub1/2, AddSub2/2
  Mux2/1 -> AddSub2/1, Register11/1
  AddSub2/1 -> Mux3/3
  MSB1/1 -> Mux3/1
  Register11/1 -> Mux3/2, MSB1/1
  AddSub/1 -> Mux1/3
  Mux3/1 -> Convert/1
  MSB/1 -> Mux2/1
  Constant1/1 -> Relational/2
  Mux1/1 -> AddSub1/1, Register10/1
  Register10/1 -> MSB/1, Mux2/2
  Relational/1 -> Mux1/1
  AddSub1/1 -> Mux2/3
  angle_in/1 -> Register9/1, Relational/1, AddSub/1

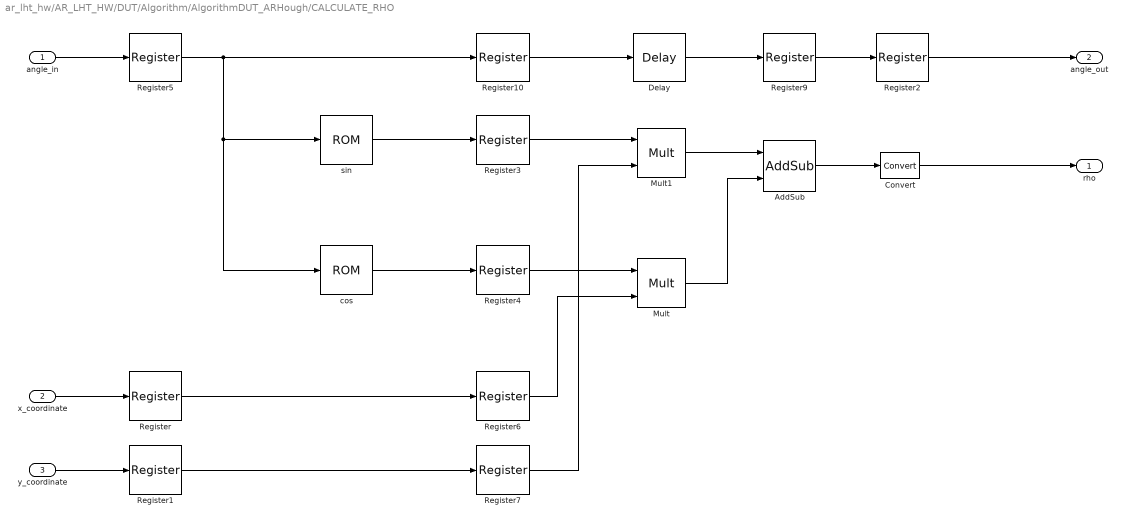
== system ar_lht_hw/AR_LHT_HW/DUT/Algorithm/AlgorithmDUT_ARHough/CALCULATE_RHO ==
  angle_in : Inport
  x_coordinate : Inport  Port=2
  y_coordinate : Inport  Port=3
  AddSub : xbsIndex_r4/AddSub  mode=Addition  use_carryin=off  use_carryout=off  en=off  latency=1  precision=Full  arith_type="Signed  (2's comp)"  n_bits=ceil(log2(maxRho)+1)  bin_pt=0  quantization="Round  (unbiased: +/- Inf)"  overflow=Saturate  use_behavioral_HDL=on  hw_selection=Fabric  pipelined=on  dbl_ovrd=off  block_type=addsub
  Convert : xbsIndex_r4/Convert  gui_display_data_type=Fixed-point  arith_type="Signed  (2's comp)"  n_bits=ceil(log2(maxRho)+1)  bin_pt=0  float_type=Single  exp_bits=8  fraction_bits=24  quantization="Round  (unbiased: +/- Inf)"  overflow=Saturate  en=off  latency=1  pipeline=off  dbl_ovrd=off  block_type=convert
  Delay : xbsIndex_r4/Delay  rst=off  infoeditControl=Selection of Reset will increase slice count due to use of real FFs and instead of SRLs  en=off  latency=3  reg_retiming=off  dbl_ovrd=off  block_type=delay
  Mult : xbsIndex_r4/Mult  precision=Full  arith_type="Signed  (2's comp)"  n_bits=16  bin_pt=14  quantization=Truncate  overflow=Wrap  en=off  latency=3  use_behavioral_HDL=off  opt=Area  use_embedded=off  optimum_pipeline=off  pipeline=on  dbl_ovrd=off  use_rpm=on  placement_style=Triangular  block_type=mult
  Mult1 : xbsIndex_r4/Mult  precision=Full  arith_type="Signed  (2's comp)"  n_bits=16  bin_pt=14  quantization=Truncate  overflow=Wrap  en=off  latency=3  use_behavioral_HDL=off  opt=Area  use_embedded=off  optimum_pipeline=off  pipeline=on  dbl_ovrd=off  use_rpm=on  placement_style=Triangular  block_type=mult
  Register{,1..7,9..10} (10 alike) : xbsIndex_r4/Register  init=0  rst=off  en=off  dbl_ovrd=off  block_type=register
  cos : xbsIndex_r4/ROM  depth=maxTheta+deltaTheta  initVector=cos(deg2rad([0:1:maxTheta]))  distributed_mem=Distributed memory  rst=off  init_reg=0  en=off  latency=0  gui_display_data_type=Fixed-point  arith_type="Signed  (2's comp)"  n_bits=14  bin_pt=13  preci_type=Single  exp_width=8  frac_width=24  optimize=Area  use_rpm=on  dbl_ovrd=off  block_type=sprom
  sin : xbsIndex_r4/ROM  depth=maxTheta+deltaTheta  initVector=sin(deg2rad([0:1:maxTheta]))  distributed_mem=Distributed memory  rst=off  init_reg=0  en=off  latency=0  gui_display_data_type=Fixed-point  arith_type="Signed  (2's comp)"  n_bits=14  bin_pt=13  preci_type=Single  exp_width=8  frac_width=24  optimize=Area  use_rpm=off  dbl_ovrd=off  block_type=sprom
  rho : Outport
  angle_out : Outport  Port=2
  wires:
  Convert/1 -> rho/1
  Register2/1 -> angle_out/1
  Register7/1 -> Mult1/2
  Register6/1 -> Mult/2
  Delay/1 -> Register9/1
  Register10/1 -> Delay/1
  Register9/1 -> Register2/1
  x_coordinate/1 -> Register/1
  Mult1/1 -> AddSub/1
  cos/1 -> Register4/1
  Mult/1 -> AddSub/2
  y_coordinate/1 -> Register1/1
  sin/1 -> Register3/1
  angle_in/1 -> Register5/1
  Register/1 -> Register6/1
  Register1/1 -> Register7/1
  Register5/1 -> sin/1, cos/1, Register10/1
  Register3/1 -> Mult1/1
  Register4/1 -> Mult/1
  AddSub/1 -> Convert/1

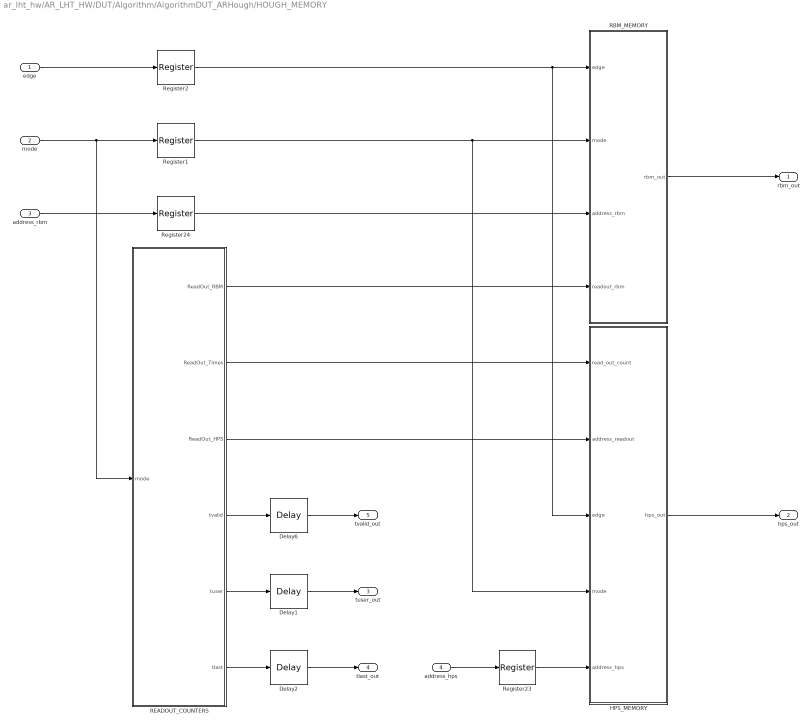
== system ar_lht_hw/AR_LHT_HW/DUT/Algorithm/AlgorithmDUT_ARHough/HOUGH_MEMORY ==
  edge : Inport
  mode : Inport  Port=2
  address_rbm : Inport  Port=3
  address_hps : Inport  Port=4
  Delay1 : xbsIndex_r4/Delay  rst=off  infoeditControl=Selection of Reset will increase slice count due to use of real FFs and instead of SRLs  en=off  latency=13  reg_retiming=off  dbl_ovrd=off  block_type=delay
  Delay2 : xbsIndex_r4/Delay  rst=off  infoeditControl=Selection of Reset will increase slice count due to use of real FFs and instead of SRLs  en=off  latency=13  reg_retiming=off  dbl_ovrd=off  block_type=delay
  Delay6 : xbsIndex_r4/Delay  rst=off  infoeditControl=Selection of Reset will increase slice count due to use of real FFs and instead of SRLs  en=off  latency=13  reg_retiming=off  dbl_ovrd=off  block_type=delay
  HPS_MEMORY : Subsystem
  RBM_MEMORY : Subsystem
  READOUT_COUNTERS : Subsystem
  Register{1..2,23..24} (4 alike) : xbsIndex_r4/Register  init=0  rst=off  en=off  dbl_ovrd=off  block_type=register
  rbm_out : Outport
  hps_out : Outport  Port=2
  tuser_out : Outport  Port=3
  tlast_out : Outport  Port=4
  tvalid_out : Outport  Port=5
  wires:
  Delay1/1 -> tuser_out/1
  RBM_MEMORY/1(rbm_out) -> rbm_out/1
  HPS_MEMORY/1(hps_out) -> hps_out/1
  Delay2/1 -> tlast_out/1
  Register23/1 -> HPS_MEMORY/5(address_hps)
  READOUT_COUNTERS/4(tvalid) -> Delay6/1
  edge/1 -> Register2/1
  READOUT_COUNTERS/3(ReadOut_HPS) -> HPS_MEMORY/2(address_readout)
  mode/1 -> READOUT_COUNTERS/1(mode), Register1/1
  address_rbm/1 -> Register24/1
  READOUT_COUNTERS/2(ReadOut_Times) -> HPS_MEMORY/1(read_out_count)
  READOUT_COUNTERS/1(ReadOut_RBM) -> RBM_MEMORY/4(readout_rbm)
  address_hps/1 -> Register23/1
  Delay6/1 -> tvalid_out/1
  Register2/1 -> RBM_MEMORY/1(edge), HPS_MEMORY/3(edge)
  READOUT_COUNTERS/5(tuser) -> Delay1/1
  Register24/1 -> RBM_MEMORY/3(address_rbm)
  Register1/1 -> HPS_MEMORY/4(mode), RBM_MEMORY/2(mode)
  READOUT_COUNTERS/6(tlast) -> Delay2/1

== system ar_lht_hw/AR_LHT_HW/DUT/Algorithm/AlgorithmDUT_ARHough/MODE_GEN ==
  tuser : Inport
  tvalid : Inport  Port=2
  Assert : xbsIndex_r4/Assert  assert_type=on  type_source=Explicitly  gui_display_data_type=Boolean  arith_type=Boolean  n_bits=16  bin_pt=14  preci_type=Single  exp_width=8  frac_width=24  assert_rate=on  rate_source=Explicitly  period=T  output_port=on  block_type=assert
  Logical : xbsIndex_r4/Logical  logical_function=NOR  inputs=2  en=off  latency=0  precision=Full  arith_type=Unsigned  n_bits=16  bin_pt=0  align_bp=on  dbl_ovrd=off  block_type=logical
  Logical1 : xbsIndex_r4/Logical  logical_function=AND  inputs=2  en=off  latency=0  precision=Full  arith_type=Unsigned  n_bits=16  bin_pt=0  align_bp=on  dbl_ovrd=off  block_type=logical
  Register13 : xbsIndex_r4/Register  init=0  rst=off  en=on  dbl_ovrd=off  block_type=register
  Register14 : xbsIndex_r4/Register  init=0  rst=off  en=on  dbl_ovrd=off  block_type=register
  mode : Outport
  wires:
  Assert/1 -> Register14/1, mode/1
  tuser/1 -> Logical1/1
  tvalid/1 -> Logical1/2, Register14/2
  Register13/1 -> Assert/1
  Logical1/1 -> Register13/2
  Logical/1 -> Register13/1
  Register14/1 -> Logical/2, Logical/1

== system ar_lht_hw/AR_LHT_HW/DUT/Algorithm/AlgorithmDUT_ARHough/POSITION_CALCULATOR ==
  tuser_in : Inport
  tvalid_in : Inport  Port=2
  Constant1 : xbsIndex_r4/Constant  const=width/2-2  gui_display_data_type=Fixed-point  arith_type=Unsigned  n_bits=ceil(log2(width/2-2))  bin_pt=0  preci_type=Single  exp_width=8  frac_width=24  explicit_period=on  period=T  equ=P=C  opselect=C  inp2=PCIN>>17  opr=+  inp1=P  carry=CIN  dbl_ovrd=off  block_type=constant
  Logical : xbsIndex_r4/Logical  logical_function=AND  inputs=2  en=off  latency=0  precision=Full  arith_type=Unsigned  n_bits=16  bin_pt=0  align_bp=on  dbl_ovrd=off  block_type=logical
  Relational : xbsIndex_r4/Relational  mode=a=b  op_type=Bool  en=on  latency=1  dbl_ovrd=off  block_type=relational
  x_counter : xbsIndex_r4/Counter  cnt_type=Count Limited  cnt_to=width/2-1  operation=Up  start_count=-width/2  cnt_by_val=1  arith_type="Signed  (2's comp)"  n_bits=ceil(log2(width/2-1)+1)  bin_pt=0  load_pin=off  rst=on  en=on  explicit_period=on  period=T  use_behavioral_HDL=on  implementation=Fabric  dbl_ovrd=off  block_type=counter
  y_counter : xbsIndex_r4/Counter  cnt_type=Count Limited  cnt_to=height/2-1  operation=Up  start_count=-height/2  cnt_by_val=1  arith_type="Signed  (2's comp)"  n_bits=ceil(log2(height/2-1)+1)  bin_pt=0  load_pin=off  rst=on  en=on  explicit_period=on  period=T  use_behavioral_HDL=on  implementation=Fabric  dbl_ovrd=off  block_type=counter
  x_coordinate : Outport
  y_coordinate : Outport  Port=2
  wires:
  tvalid_in/1 -> Relational/3, x_counter/2, Logical/2
  Relational/1 -> Logical/1
  Logical/1 -> y_counter/2
  x_counter/1 -> x_coordinate/1, Relational/1
  y_counter/1 -> y_coordinate/1
  tuser_in/1 -> x_counter/1, y_counter/1
  Constant1/1 -> Relational/2

== system ar_lht_hw/AR_LHT_HW/DUT/Algorithm/AlgorithmDUT_ARHough/Registers ==
  In1 : Inport
  Register5 : xbsIndex_r4/Register  init=0  rst=off  en=off  dbl_ovrd=off  block_type=register
  Register7 : xbsIndex_r4/Register  init=0  rst=off  en=off  dbl_ovrd=off  block_type=register
  Out1 : Outport
  wires:
  Register7/1 -> Out1/1
  In1/1 -> Register5/1
  Register5/1 -> Register7/1

== system ar_lht_hw/AR_LHT_HW/DUT/Algorithm/AlgorithmDUT_ARHough/Registers1 ==
  In1 : Inport
  Register{1..7} (7 alike) : xbsIndex_r4/Register  init=0  rst=off  en=off  dbl_ovrd=off  block_type=register
  Out1 : Outport
  wires:
  Register6/1 -> Out1/1
  Register4/1 -> Register3/1
  Register3/1 -> Register2/1
  Register2/1 -> Register1/1
  Register7/1 -> Register6/1
  In1/1 -> Register4/1
  Register5/1 -> Register7/1
  Register1/1 -> Register5/1

== system ar_lht_hw/AR_LHT_HW/DUT/Algorithm/AlgorithmDUT_ARHough/Registers2 ==
  In1 : Inport
  Register1 : xbsIndex_r4/Register  init=0  rst=off  en=off  dbl_ovrd=off  block_type=register
  Register5 : xbsIndex_r4/Register  init=0  rst=off  en=off  dbl_ovrd=off  block_type=register
  Register7 : xbsIndex_r4/Register  init=0  rst=off  en=off  dbl_ovrd=off  block_type=register
  Out1 : Outport
  wires:
  Register1/1 -> Register5/1
  Register5/1 -> Register7/1
  In1/1 -> Register1/1
  Register7/1 -> Out1/1

== system ar_lht_hw/AR_LHT_HW/DUT/Algorithm/AlgorithmDUT_ARHough/Registers3 ==
  In1 : Inport
  Register1 : xbsIndex_r4/Register  init=0  rst=off  en=off  dbl_ovrd=off  block_type=register
  Register5 : xbsIndex_r4/Register  init=0  rst=off  en=off  dbl_ovrd=off  block_type=register
  Register7 : xbsIndex_r4/Register  init=0  rst=off  en=off  dbl_ovrd=off  block_type=register
  Out1 : Outport
  wires:
  Register1/1 -> Register5/1
  Register7/1 -> Out1/1
  In1/1 -> Register1/1
  Register5/1 -> Register7/1

== system ar_lht_hw/AR_LHT_HW/DUT/Algorithm/AlgorithmDUT_ARHough/Registers4 ==
  In1 : Inport
  Register1 : xbsIndex_r4/Register  init=0  rst=off  en=off  dbl_ovrd=off  block_type=register
  Register5 : xbsIndex_r4/Register  init=0  rst=off  en=off  dbl_ovrd=off  block_type=register
  Register7 : xbsIndex_r4/Register  init=0  rst=off  en=off  dbl_ovrd=off  block_type=register
  Out1 : Outport
  wires:
  Register7/1 -> Out1/1
  In1/1 -> Register1/1
  Register5/1 -> Register7/1
  Register1/1 -> Register5/1

== system ar_lht_hw/AR_LHT_HW/DUT/Algorithm/AlgorithmDUT_ARHough/Registers5 ==
  In1 : Inport
  Register1 : xbsIndex_r4/Register  init=0  rst=off  en=off  dbl_ovrd=off  block_type=register
  Register5 : xbsIndex_r4/Register  init=0  rst=off  en=off  dbl_ovrd=off  block_type=register
  Register7 : xbsIndex_r4/Register  init=0  rst=off  en=off  dbl_ovrd=off  block_type=register
  Out1 : Outport
  wires:
  Register1/1 -> Register5/1
  Register5/1 -> Register7/1
  In1/1 -> Register1/1
  Register7/1 -> Out1/1

== system ar_lht_hw/AR_LHT_HW/DUT/Algorithm/AlgorithmDUT_ARHough/Registers6 ==
  In1 : Inport
  Register5 : xbsIndex_r4/Register  init=0  rst=off  en=off  dbl_ovrd=off  block_type=register
  Register7 : xbsIndex_r4/Register  init=0  rst=off  en=off  dbl_ovrd=off  block_type=register
  Out1 : Outport
  wires:
  Register5/1 -> Register7/1
  In1/1 -> Register5/1
  Register7/1 -> Out1/1

== system ar_lht_hw/AR_LHT_HW/DUT/Algorithm/AlgorithmDUT_ARHough/Registers7 ==
  In1 : Inport
  Register{1..7} (7 alike) : xbsIndex_r4/Register  init=0  rst=off  en=off  dbl_ovrd=off  block_type=register
  Out1 : Outport
  wires:
  Register6/1 -> Out1/1
  Register1/1 -> Register5/1
  Register5/1 -> Register7/1
  In1/1 -> Register4/1
  Register7/1 -> Register6/1
  Register2/1 -> Register1/1
  Register3/1 -> Register2/1
  Register4/1 -> Register3/1

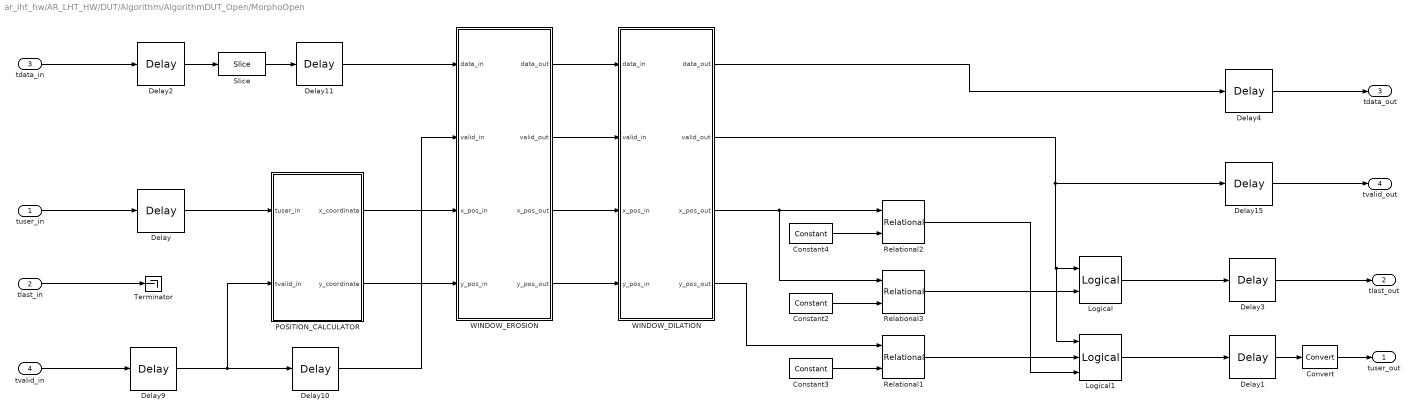
== system ar_lht_hw/AR_LHT_HW/DUT/Algorithm/AlgorithmDUT_Open/MorphoOpen ==
  tuser_in : Inport
  tlast_in : Inport  Port=2
  tdata_in : Inport  Port=3
  tvalid_in : Inport  Port=4
  Constant2 : xbsIndex_r4/Constant  const=width/2  gui_display_data_type=Fixed-point  arith_type=Unsigned  n_bits=32  bin_pt=0  preci_type=Single  exp_width=8  frac_width=24  explicit_period=on  period=T  equ=P=C  opselect=C  inp2=PCIN>>17  opr=+  inp1=P  carry=CIN  dbl_ovrd=off  block_type=constant
  Constant3 : xbsIndex_r4/Constant  const=-height/2+1  gui_display_data_type=Fixed-point  arith_type=Signed (2's comp)  n_bits=32  bin_pt=0  preci_type=Single  exp_width=8  frac_width=24  explicit_period=on  period=T  equ=P=C  opselect=C  inp2=PCIN>>17  opr=+  inp1=P  carry=CIN  dbl_ovrd=off  block_type=constant
  Constant4 : xbsIndex_r4/Constant  const=-width/2+1  gui_display_data_type=Fixed-point  arith_type=Signed (2's comp)  n_bits=32  bin_pt=0  preci_type=Single  exp_width=8  frac_width=24  explicit_period=on  period=T  equ=P=C  opselect=C  inp2=PCIN>>17  opr=+  inp1=P  carry=CIN  dbl_ovrd=off  block_type=constant
  Convert : xbsIndex_r4/Convert  gui_display_data_type=Fixed-point  arith_type=Unsigned  n_bits=1  bin_pt=0  float_type=Single  exp_bits=8  fraction_bits=24  quantization=Truncate  overflow=Wrap  en=off  latency=0  pipeline=off  dbl_ovrd=off  block_type=convert
  Delay{,1..4,9..11,15} (9 alike) : xbsIndex_r4/Delay  rst=off  infoeditControl=Selection of Reset will increase slice count due to use of real FFs and instead of SRLs  en=off  latency=1  reg_retiming=off  dbl_ovrd=off  block_type=delay
  Logical : xbsIndex_r4/Logical  logical_function=AND  inputs=2  en=off  latency=0  precision=Full  arith_type=Unsigned  n_bits=16  bin_pt=0  align_bp=on  dbl_ovrd=off  block_type=logical
  Logical1 : xbsIndex_r4/Logical  logical_function=AND  inputs=3  en=off  latency=0  precision=Full  arith_type=Unsigned  n_bits=16  bin_pt=0  align_bp=on  dbl_ovrd=off  block_type=logical
  POSITION_CALCULATOR : Subsystem
  Relational1 : xbsIndex_r4/Relational  mode=a=b  op_type=Bool  en=off  latency=0  dbl_ovrd=off  block_type=relational
  Relational2 : xbsIndex_r4/Relational  mode=a=b  op_type=Bool  en=off  latency=0  dbl_ovrd=off  block_type=relational
  Relational3 : xbsIndex_r4/Relational  mode=a=b  op_type=Bool  en=off  latency=0  dbl_ovrd=off  block_type=relational
  Slice : xbsIndex_r4/Slice  nbits=1  boolean_output=on  mode=Two Bit Locations  bit1=0  base1=LSB of Input  bit0=0  base0=LSB of Input  dbl_ovrd=off  block_type=slice
  Terminator : Terminator
  WINDOW_DILATION : Subsystem
  WINDOW_EROSION : Subsystem
  tuser_out : Outport
  tlast_out : Outport  Port=2
  tdata_out : Outport  Port=3
  tvalid_out : Outport  Port=4
  wires:
  Delay11/1 -> WINDOW_EROSION/1(data_in)
  Slice/1 -> Delay11/1
  tvalid_in/1 -> Delay9/1
  Delay2/1 -> Slice/1
  Convert/1 -> tuser_out/1
  Constant2/1 -> Relational3/2
  Constant3/1 -> Relational1/2
  Logical1/1 -> Delay1/1
  Logical/1 -> Delay3/1
  Relational1/1 -> Logical1/2
  Relational3/1 -> Logical/2
  Delay1/1 -> Convert/1
  Delay/1 -> POSITION_CALCULATOR/1(tuser_in)
  Delay3/1 -> tlast_out/1
  tuser_in/1 -> Delay/1
  tdata_in/1 -> Delay2/1
  Delay4/1 -> tdata_out/1
  Relational2/1 -> Logical1/3
  POSITION_CALCULATOR/1(x_coordinate) -> WINDOW_EROSION/3(x_pos_in)
  POSITION_CALCULATOR/2(y_coordinate) -> WINDOW_EROSION/4(y_pos_in)
  tlast_in/1 -> Terminator/1
  Delay9/1 -> POSITION_CALCULATOR/2(tvalid_in), Delay10/1
  Delay10/1 -> WINDOW_EROSION/2(valid_in)
  Delay15/1 -> tvalid_out/1
  Constant4/1 -> Relational2/2
  WINDOW_EROSION/4(y_pos_out) -> WINDOW_DILATION/4(y_pos_in)
  WINDOW_EROSION/3(x_pos_out) -> WINDOW_DILATION/3(x_pos_in)
  WINDOW_EROSION/2(valid_out) -> WINDOW_DILATION/2(valid_in)
  WINDOW_EROSION/1(data_out) -> WINDOW_DILATION/1(data_in)
  WINDOW_DILATION/3(x_pos_out) -> Relational3/1, Relational2/1
  WINDOW_DILATION/4(y_pos_out) -> Relational1/1
  WINDOW_DILATION/2(valid_out) -> Delay15/1, Logical1/1, Logical/1
  WINDOW_DILATION/1(data_out) -> Delay4/1
